simulink model "IEEE9_16b_central"  (R2020a)
settings: Solver=FixedStepAuto  StartTime=0.0  StopTime=5  FixedStep=1/1200/30  MaxStep=1e-4  RelTol=1e-3
undefined symbols (not defined in the file or in its folder): k
libraries: powerlib x33, powerlib_meascontrol x27, simulink_extras x24, dspsigops x6, sps_avr x3
(part 1 of 2)
settings Model: Creator=Pankaj  LastModifiedBy=ahmed
settings DataIOCC: ReturnWorkspaceOutputs=off  Refine=100
settings DebuggingCC: UnconnectedInputMsg=none  UnconnectedOutputMsg=none  UnconnectedLineMsg=none  ArithmeticOperatorsInVariantConditions=warning
settings SFSimCC: SimUseLocalCustomCode=off  CustomCodeUndefinedFunction=UseInterfaceOnly
settings RTWCC: RTWUseLocalCustomCode=off
settings CodeAppCC: StateflowObjectComments=on
settings SimscapeCC: SimscapeNormalizeSystem=off

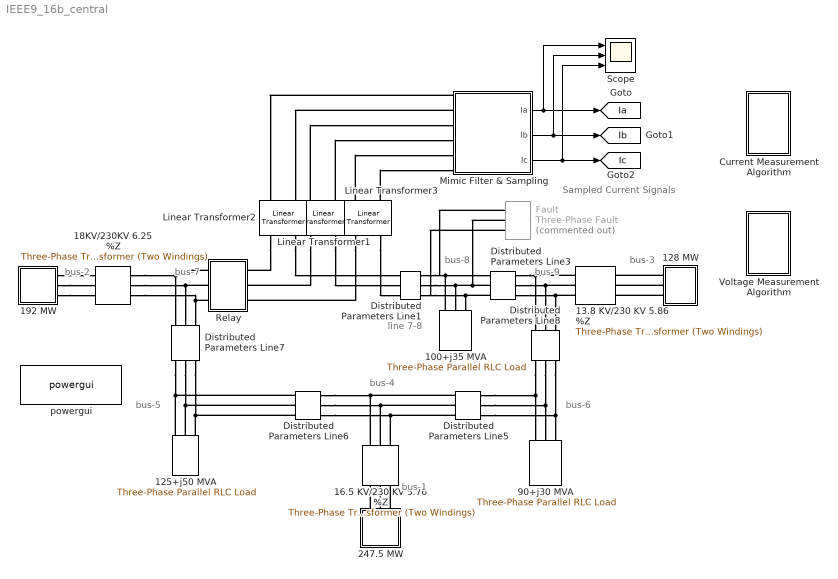
== system IEEE9_16b_central ==
  note: bus-2
  note: bus-7
  note: bus-8
  note: bus-9
  note: bus-1
  note: bus-3
  note: bus-4
  note: bus-6
  note: bus-5
  note: line 7-8
  note: Sampled Current Signals
  100+j35 MVA : powerlib/Elements/Three-Phase Parallel RLC Load  LConnTagsString=A|B|C  Configuration=Y (grounded)  NominalVoltage=(230000)*0.993698  Vabc=[1e3 1e3 1e3]  Vabcp=[1e3 1e3 1e3]  NominalFrequency=60  UnbalancedPower=off  ActivePower=100e6  InductivePower=35e6  CapacitivePower=0  Pabc=[10e3 9e3 11e3]  QLabc=[100 90 110]  QCabc=[100 90 110]  Pabcp=[10e3 9e3 11e3]  QLabcp=[100 90 110]  QCabcp=[100 90 110]  Measurements=None  LoadType=constant PQ
  125+j50 MVA : powerlib/Elements/Three-Phase Parallel RLC Load  LConnTagsString=A|B|C  Configuration=Y (grounded)  NominalVoltage=(223027)*1  Vabc=[1e3 1e3 1e3]  Vabcp=[1e3 1e3 1e3]  NominalFrequency=60  UnbalancedPower=off  ActivePower=125e6  InductivePower=50e6  CapacitivePower=0  Pabc=[10e3 9e3 11e3]  QLabc=[100 90 110]  QCabc=[100 90 110]  Pabcp=[10e3 9e3 11e3]  QLabcp=[100 90 110]  QCabcp=[100 90 110]  Measurements=None  LoadType=constant PQ
  128 MW : Subsystem
  13.8 KV/230 KV 5.86 %Z : powerlib/Elements/Three-Phase Transformer (Two Windings)  Winding1Connection=Yg  Winding2Connection=Yg  CoreType=Three single-phase transformers  SetSaturation=off  Hysteresis=off  DataFile='hysteresis'  SetInitialFlux=off  Measurements=None  UNITS=pu  NominalPower=[ 100e6 , 60 ]  Winding1=[13.8e3 , 1e-6 , 0 ]  Winding2=[ 230e3 , 1e-6, 0.0586 ]  Rm=500  Lm=500  L0=0.5  Saturation=[ 0,0 ; 0.0024,1.2 ; 1.0,1.52 ]  InitialFluxes=[ 0.8 , -0.8 , 0.7 ]  BreakLoop=off  DiscreteSolver=Trapezoidal iterative  DataType=off  TransfoNumber=1
  "16.5 KV/230 KV 5.76 %Z     " : powerlib/Elements/Three-Phase Transformer (Two Windings)  Winding1Connection=Yg  Winding2Connection=Yg  CoreType=Three single-phase transformers  SetSaturation=off  Hysteresis=off  DataFile='hysteresis'  SetInitialFlux=off  Measurements=None  UNITS=pu  NominalPower=[ 100e6 , 60 ]  Winding1=[16.5e3 , 1e-6, 0 ]  Winding2=[ 230e3 ,1e-6, 0.0576 ]  Rm=500  Lm=500  L0=0.5  Saturation=[ 0,0 ; 0.0024,1.2 ; 1.0,1.52 ]  InitialFluxes=[ 0.8 , -0.8 , 0.7 ]  BreakLoop=off  DiscreteSolver=Trapezoidal iterative  DataType=off  TransfoNumber=1
  18KV/230KV 6.25 %Z : powerlib/Elements/Three-Phase Transformer (Two Windings)  Winding1Connection=Yg  Winding2Connection=Yg  CoreType=Three single-phase transformers  SetSaturation=off  Hysteresis=off  DataFile='hysteresis'  SetInitialFlux=off  Measurements=None  UNITS=pu  NominalPower=[ 100e6 , 60 ]  Winding1=[ 18e3 , 1e-6 , 0]  Winding2=[ 230e3 , 1e-6, 0.0625 ]  Rm=500  Lm=500  L0=0.5  Saturation=[ 0,0 ; 0.0024,1.2 ; 1.0,1.52 ]  InitialFluxes=[ 0.8 , -0.8 , 0.7 ]  BreakLoop=off  DiscreteSolver=Trapezoidal iterative  DataType=off  TransfoNumber=1
  192 MW : Subsystem
  247.5 MW : Subsystem
  90+j30 MVA : powerlib/Elements/Three-Phase Parallel RLC Load  LConnTagsString=A|B|C  Configuration=Y (grounded)  NominalVoltage=(226177)*0.999999  Vabc=[1e3 1e3 1e3]  Vabcp=[1e3 1e3 1e3]  NominalFrequency=60  UnbalancedPower=off  ActivePower=90e6  InductivePower=30e6  CapacitivePower=0  Pabc=[10e3 9e3 11e3]  QLabc=[100 90 110]  QCabc=[100 90 110]  Pabcp=[10e3 9e3 11e3]  QLabcp=[100 90 110]  QCabcp=[100 90 110]  Measurements=None  LoadType=constant PQ
  Current Measurement Algorithm : Subsystem
  Distributed Parameters Line1 : powerlib/Elements/Distributed Parameters Line  Phases=3  Frequency=60  Resistance=[0.044965 0.11241]  Inductance="[1.01e-3  2.02e-3]"  Capacitance=[12.74e-9 7.751e-9]  Length=100  x1=[-0.000416666666666667 3.05242528703213e-10 0 0;-0.000388888888888889 3.05500631439883e-10 0 0;-0.000361111111111111 3.05725232589637e-10 75589.8043140482 -217739.673406231;-0.000333333333333333 3.05916307522428e-10 77865.7774864176 -216936.173033532;-0.000305555555555556 3.06073835284735e-10 80133.2117988181 -216108.883164811;-0.000277777777777778 3.06197798601864e-10 82391.8586015257 -215257.894521725;-0.00025 3.06288183879841e-10 84641.4702084657 -214383.30042477;-0.000222222222222222 3.06344981206902e-10 86881.7999243747 -213485.196783042;-0.000194444444444444 3.06368184354579e-10 89112.6020718531 -212563.682083727;-0.000166666666666667 3.06357790778386e-10 91333.6320183066 -211618.857381298;-0.000138888888888889 3.06313801618096e-10 93544.6462027728 -210650.826286428;-0.000111111111111111 3.06236221697615e-10 95745.4021626305 -209659.694954637;-8.33333333333333e-05 3.06125059524457e-10 97935.6585601885 -208645.572074645;-5.55555555555556e-05 3.05980327288806e-10 100115.175209151 -207608.568856452;-2.77777777777778e-05 3.05802040862183e-10 102283.713100956 -206548.799019148]  x2=[-0.000416666666666667 1.02171489544743e-10 0 0;-0.000388888888888889 1.0125535769788e-10 0 0;-0.000361111111111111 1.00328122060001e-10 65357.6959924733 -218991.76000131;-0.000333333333333333 9.93898843129427e-11 67647.34161361 -218295.340188402;-0.000305555555555556 9.84407473450475e-11 69929.5689414224 -217574.981831478;-0.000277777777777778 9.74808152398795e-11 72204.1277039659 -216830.763925948;-0.00025 9.65101932648115e-11 74470.76847024 -216062.768083693;-0.000222222222222222 9.55289878594811e-11 76729.2426775421 -215271.078524112;-0.000194444444444444 9.45373066241179e-11 78979.3026587246 -214455.782064886;-0.000166666666666667 9.35352583077448e-11 81220.7016693547 -213616.96811246;-0.000138888888888889 9.25229527962518e-11 83453.1939147727 -212754.728652235;-0.000111111111111111 9.15005011003457e-11 85676.5345770459 -211869.158238486;-8.33333333333333e-05 9.0468015343377e-11 87890.4798418159 -210960.353983988;-5.55555555555556e-05 8.94256087490441e-11 90094.7869250356 -210028.415549369;-2.77777777777778e-05 8.83733956289768e-11 92289.214099593 -209073.445132179]  x3=[-0.000416666666666667 1.88047725229952e-12 0 0;-0.000388888888888889 1.85577565108302e-12 0 0;-0.000361111111111111 1.83087054315368e-12 150.014670555124 -522.196921384387;-0.000333333333333333 1.80576465963726e-12 155.474780219226 -520.59737046614;-0.000305555555555556 1.78046075367679e-12 160.917840321636 -518.940730179622;-0.000277777777777778 1.75496160013071e-12 166.343253969475 -517.227182194109;-0.00025 1.72926999526855e-12 171.750426204999 -515.456914419448;-0.000222222222222222 1.70338875646432e-12 177.138764070837 -513.63012098545;-0.000194444444444444 1.67732072188749e-12 182.507676675023 -511.7470022206;-0.000166666666666667 1.65106875019181e-12 187.856575255787 -509.807764630092;-0.000138888888888889 1.62463572020183e-12 193.184873246123 -507.812620873181;-0.000111111111111111 1.59802453059714e-12 198.491986338112 -505.761789739863;-8.33333333333333e-05 1.57123809959458e-12 203.777332546997 -503.655496126883;-5.55555555555556e-05 1.54427936462815e-12 209.040332275007 -501.493971013071;-2.77777777777778e-05 1.51715128202694e-12 214.280408374913 -499.277451434014]  x4=[-0.000416666666666667 -8.7518100237193e-13 0 0;-0.000388888888888889 -8.47376987953706e-13 0 0;-0.000361111111111111 -8.19480049099682e-13 240.406666770988 -1044.04487087356;-0.000333333333333333 -7.91493245023573e-13 251.326459490831 -1041.47013077654;-0.000305555555555556 -7.6341964479383e-13 262.218691432199 -1038.78118174338;-0.000277777777777778 -7.35262326997077e-13 273.082168139116 -1035.97831864764;-0.00025 -7.07024379400516e-13 283.915698308939 -1033.06184885485;-0.000222222222222222 -6.78708898613313e-13 294.718093923004 -1030.03209218878;-0.000194444444444444 -6.50318989747023e-13 305.488170376899 -1026.88938089639;-0.000166666666666667 -6.21857766075078e-13 316.224746610374 -1023.6340596114;-0.000138888888888889 -5.93328348691383e-13 326.926645236854 -1020.26648531647;-0.000111111111111111 -5.64733866168052e-13 337.592692672555 -1016.78702730406;-8.33333333333333e-05 -5.36077454212322e-13 348.221719265181 -1013.19606713596;-5.55555555555556e-05 -5.07362255322695e-13 358.812559422187 -1009.49399860142;-2.77777777777778e-05 -4.78591418444318e-13 369.364051738602 -1005.68122767396]  x5=0.000395689524753941  V1=[5.416e-10 2.305e+05 2.305e+05;377 377 377;2.885 0.3359 -1.235]  V2=[2.789e-10 2.285e+05 2.285e+05;377 377 377;2.728 0.2916 -1.279]  I1=[3.179e-12 542 542;377 377 377;-1.76 0.2811 -1.29]  I2=[4.124e-12 1072 1072;377 377 377;1.614 0.2282 -1.343]  nHarmo=1  Measurements=None
  Distributed Parameters Line3 : powerlib/Elements/Distributed Parameters Line  Phases=3  Frequency=60  Resistance=[ 0.062951 0.15737]  Inductance="[ 1.414e-3  3.53e-3]"  Capacitance=[12.74e-9 7.751e-9]  Length=100  x1=[-0.000527777777777778 1.05722988233672e-10 0 0;-0.0005 1.04852263851676e-10 0 0;-0.000472222222222222 1.03970041237372e-10 0 0;-0.000444444444444444 1.0307641713641e-10 58446.7641257665 -220936.637648747;-0.000416666666666667 1.02171489544743e-10 60757.1549979699 -220312.481147461;-0.000388888888888889 1.0125535769788e-10 63060.8831634568 -219664.164899921;-0.000361111111111111 1.00328122060001e-10 65357.6959924733 -218991.76000131;-0.000333333333333333 9.93898843129427e-11 67647.34161361 -218295.340188402;-0.000305555555555556 9.84407473450475e-11 69929.5689414224 -217574.981831478;-0.000277777777777778 9.74808152398795e-11 72204.1277039659 -216830.763925948;-0.00025 9.65101932648115e-11 74470.76847024 -216062.768083693;-0.000222222222222222 9.55289878594811e-11 76729.2426775421 -215271.078524112;-0.000194444444444444 9.45373066241179e-11 78979.3026587246 -214455.782064886;-0.000166666666666667 9.35352583077448e-11 81220.7016693547 -213616.96811246;-0.000138888888888889 9.25229527962518e-11 83453.1939147727 -212754.728652235;-0.000111111111111111 9.15005011003457e-11 85676.5345770459 -211869.158238486;-8.33333333333333e-05 9.0468015343377e-11 87890.4798418159 -210960.353983988;-5.55555555555556e-05 8.94256087490441e-11 90094.7869250356 -210028.415549369;-2.77777777777778e-05 8.83733956289768e-11 92289.214099593 -209073.445132179]  x2=[-0.000527777777777778 9.13415239263644e-11 0 0;-0.0005 9.12184788255193e-11 0 0;-0.000472222222222222 9.10854305905322e-11 0 0;-0.000444444444444444 9.09423938116413e-11 67569.0569929193 -221221.006139122;-0.000416666666666667 9.07893841744413e-11 69881.9252697332 -220501.30792954;-0.000388888888888889 9.06264184581633e-11 72187.1302059435 -219757.42926672;-0.000361111111111111 9.04535145338344e-11 74484.4190098517 -218989.451725339;-0.000333333333333333 9.02706913623184e-11 76773.5397578524 -218197.45952279;-0.000305555555555556 9.00779689922363e-11 79054.2414220595 -217381.539509942;-0.000277777777777778 8.98753685577677e-11 81326.2738978343 -216541.78116162;-0.00025 8.96629122763335e-11 83589.3880312124 -215678.276566789;-0.000222222222222222 8.9440623446159e-11 85843.3356462261 -214791.120418459;-0.000194444444444444 8.92085264437193e-11 88087.8695721197 -213880.4100033;-0.000166666666666667 8.89666467210664e-11 90322.7436704547 -212946.24519097;-0.000138888888888889 8.87150108030376e-11 92547.7128621014 -211988.72842317;-0.000111111111111111 8.84536462843469e-11 94762.5331541149 -211007.964702401;-8.33333333333333e-05 8.81825818265591e-11 96966.9616664913 -210004.06158046;-5.55555555555556e-05 8.79018471549467e-11 99160.7566588026 -208977.129146636;-2.77777777777778e-05 8.76114730552299e-11 101343.677556706 -207927.280015642]  x3=[-0.000527777777777778 -5.71619859169204e-13 0 0;-0.0005 -5.80597990208738e-13 0 0;-0.000472222222222222 -5.89512452135901e-13 0 0;-0.000444444444444444 -5.98362267379486e-13 134.783300599734 -836.294175870902;-0.000416666666666667 -6.07146465457522e-13 143.533396667207 -834.836905447173;-0.000388888888888889 -6.15864083083703e-13 152.267752680261 -833.288085749006;-0.000361111111111111 -6.24514164273016e-13 160.985410818333 -831.647886621933;-0.000333333333333333 -6.33095760446581e-13 169.685415091968 -829.916487932272;-0.000305555555555556 -6.41607930535672e-13 178.366811447656 -828.0940795474;-0.000277777777777778 -6.50049741084917e-13 187.028647872459 -826.180861314934;-0.00025 -6.58420266354656e-13 195.669974498401 -824.177043040813;-0.000222222222222222 -6.66718588422468e-13 204.289843706639 -822.082844466291;-0.000194444444444444 -6.74943797283823e-13 212.887310231377 -819.898495243842;-0.000166666666666667 -6.83094990951881e-13 221.461431263526 -817.624234911973;-0.000138888888888889 -6.91171275556401e-13 230.011266554094 -815.260312868959;-0.000111111111111111 -6.99171765441763e-13 238.535878517293 -812.806988345489;-8.33333333333333e-05 -7.07095583264095e-13 247.034332333357 -810.264530376245;-5.55555555555556e-05 -7.14941860087479e-13 255.505696051058 -807.633217770394;-2.77777777777778e-05 -7.22709735479242e-13 263.949040689898 -804.913339081016]  x4=[-0.000527777777777778 6.12064546598544e-13 0 0;-0.0005 6.08521806486011e-13 0 0;-0.000472222222222222 6.04912335099979e-13 0 0;-0.000444444444444444 6.01236528259661e-13 132.734580460085 -502.248002708346;-0.000416666666666667 5.974947890587e-13 137.986709125664 -500.830491731963;-0.000388888888888889 5.93687527820964e-13 143.223705993618 -499.358059048314;-0.000361111111111111 5.89815162055552e-13 148.444996768225 -497.830866126237;-0.000333333333333333 5.85878116411009e-13 153.650008876114 -496.249080439645;-0.000305555555555556 5.81876822628754e-13 158.838171529051 -494.612875449165;-0.000277777777777778 5.77811719495742e-13 164.008915786537 -492.92243058311;-0.00025 5.73683252796342e-13 169.161674618194 -491.177931217812;-0.000222222222222222 5.69491875263449e-13 174.29588296595 -489.379568657283;-0.000194444444444444 5.65238046528844e-13 179.410977806003 -487.527540112244;-0.000166666666666667 5.60922233072783e-13 184.506398210562 -485.622048678496;-0.000138888888888889 5.56544908172847e-13 189.581585409359 -483.663303314648;-0.000111111111111111 5.52106551852038e-13 194.635982850925 -481.651518819201;-8.33333333333333e-05 5.47607650826144e-13 199.669036263624 -479.586915806996;-5.55555555555556e-05 5.43048698450359e-13 204.680193716431 -477.469720685019;-2.77777777777778e-05 5.38430194665186e-13 209.66890567946 -475.300165627575]  x5=0.000523077718890797  V1=[2.541e-10 2.285e+05 2.285e+05;377 377 377;2.713 0.2668 -1.304]  V2=[4.31e-10 2.313e+05 2.313e+05;377 377 377;2.564 0.3044 -1.266]  I1=[1.418e-12 846 846;377 377 377;1.513 0.1676 -1.403]  I2=[2.062e-12 520.4 520.5;377 377 377;-2.991 0.2668 -1.304]  nHarmo=1  Measurements=None
  Distributed Parameters Line5 : powerlib/Elements/Distributed Parameters Line  Phases=3  Frequency=60  Resistance=[ 0.08993 0.224825]  Inductance="[ 1.29e-3  3.22e-3]"  Capacitance=[12.74e-9 7.751e-9]  Length=100  x1=[-0.0005 1.84418084980096e-10 59301.0004761159 -221128.521904105;-0.000472222222222222 1.86482822406443e-10 61613.3539298093 -220495.408761845;-0.000444444444444444 1.88527109889844e-10 63918.9507849249 -219838.115813256;-0.000416666666666667 1.90550723251138e-10 66217.5382067858 -219156.715137918;-0.000388888888888889 1.92553440578315e-10 68508.8641293785 -218451.281459093;-0.000361111111111111 1.94535042250854e-10 70792.6772829948 -217721.892135534;-0.000333333333333333 1.96495310963798e-10 73068.7272217859 -216968.627152999;-0.000305555555555556 1.98434031751595e-10 75336.7643512275 -216191.569115483;-0.000277777777777778 2.00350992011662e-10 77596.5399554898 -215390.803236157;-0.00025 2.02245981527704e-10 79847.8062247124 -214566.417328021;-0.000222222222222222 2.04118792492767e-10 82090.3162821795 -213718.501794282;-0.000194444444444444 2.05969219532023e-10 84323.8242113925 -212847.149618432;-0.000166666666666667 2.07797059725295e-10 86548.0850830376 -211952.456354057;-0.000138888888888889 2.09602112629309e-10 88762.8549818451 -211034.520114356;-0.000111111111111111 2.11384180299671e-10 90967.8910333373 -210093.441561382;-8.33333333333333e-05 2.13143067312581e-10 93162.9514304628 -209129.323895003;-5.55555555555556e-05 2.14878580786255e-10 95347.7954601129 -208142.272841585;-2.77777777777778e-05 2.16590530402085e-10 97522.1835295188 -207132.3966424]  x2=[-0.0005 1.973914942299e-10 47829.0767997227 -221055.102399272;-0.000472222222222222 1.97930112644823e-10 50141.2903619321 -220542.12557881;-0.000444444444444444 1.98447025792425e-10 52448.0053666123 -220004.963828994;-0.000416666666666667 1.98942176987354e-10 54748.9688564689 -219443.676055664;-0.000388888888888889 1.99415511930702e-10 57043.9285049254 -218858.323810348;-0.000361111111111111 1.99866978715958e-10 59332.6326437948 -218248.971283518;-0.000333333333333333 2.00296527834702e-10 61614.8302908768 -217615.685297545;-0.000305555555555556 2.00704112182032e-10 63890.2711774814 -216958.535299372;-0.000277777777777778 2.01089687061731e-10 66158.7057758734 -216277.593352903;-0.00025 2.0145321019117e-10 68419.8853266363 -215572.934131097;-0.000222222222222222 2.01794641705939e-10 70673.5618659511 -214844.634907777;-0.000194444444444444 2.02113944164227e-10 72919.4882527886 -214092.77554916;-0.000166666666666667 2.02411082550919e-10 75157.4181960113 -213317.438505097;-0.000138888888888889 2.02686024281445e-10 77387.1062813816 -212518.708800034;-0.000111111111111111 2.02938739205344e-10 79608.3079984748 -211696.674023683;-8.33333333333333e-05 2.03169199609578e-10 81820.7797674918 -210851.42432142;-5.55555555555556e-05 2.03377380221565e-10 84024.278965971 -209983.052384401;-2.77777777777778e-05 2.03563258211957e-10 86218.563955394 -209091.653439394]  x3=[-0.0005 1.45931914328997e-12 89.8864515456847 -468.322639248616;-0.000472222222222222 1.46185650921508e-12 94.7856956152835 -467.355690941637;-0.000444444444444444 1.46423356610033e-12 99.6745453652203 -466.337491816527;-0.000416666666666667 1.46645005327464e-12 104.552464678028 -465.268153530294;-0.000388888888888889 1.46850572767522e-12 109.418918634884 -464.14779334793;-0.000361111111111111 1.47040036387421e-12 114.273373574273 -462.976534129555;-0.000333333333333333 1.47213375410339e-12 119.115297150506 -461.754504316942;-0.000305555555555556 1.47370570827699e-12 123.944158392098 -460.48183791943;-0.000277777777777778 1.47511605401253e-12 128.75942776 -459.158674499231;-0.00025 1.4763646366497e-12 133.56057720566 -457.785159156126;-0.000222222222222222 1.47745131926734e-12 138.347080228939 -456.36144251155;-0.000194444444444444 1.47837598269846e-12 143.118411935841 -454.887680692075;-0.000166666666666667 1.4791385255433e-12 147.874049096077 -453.364035312295;-0.000138888888888889 1.47973886418043e-12 152.613470200439 -451.790673457095;-0.000111111111111111 1.48017693277596e-12 157.336155517997 -450.167767663332;-8.33333333333333e-05 1.48045268329074e-12 162.041587153085 -448.495495900915;-5.55555555555556e-05 1.48056608548561e-12 166.729249102099 -446.774041553287;-2.77777777777778e-05 1.48051712692474e-12 171.398627310082 -445.003593397318]  x4=[-0.0005 -9.64211279668315e-13 134.813064300476 -917.533563496279;-0.000472222222222222 -9.64297994881882e-13 144.413854297421 -916.071516812538;-0.000444444444444444 -9.64278963953659e-13 153.998807687847 -914.509012563791;-0.000416666666666667 -9.64154188970602e-13 163.5668733736 -912.846222096237;-0.000388888888888889 -9.63923683615695e-13 173.117002108457 -911.083327753587;-0.000361111111111111 -9.63587473166446e-13 182.648146613182 -909.220522857074;-0.000333333333333333 -9.63145594492122e-13 192.159261690373 -907.258011684245;-0.000305555555555556 -9.62598096049696e-13 201.649304339081 -905.196009446567;-0.000277777777777778 -9.61945037878544e-13 211.117233869188 -903.03474226582;-0.00025 -9.61186491593854e-13 220.562012015526 -900.774447149308;-0.000222222222222222 -9.60322540378773e-13 229.982603051738 -898.415371963861;-0.000194444444444444 -9.59353278975288e-13 239.377973903858 -895.957775408657;-0.000166666666666667 -9.58278813673834e-13 248.747094263594 -893.401926986852;-0.000138888888888889 -9.57099262301641e-13 258.088936701319 -890.748106976029;-0.000111111111111111 -9.55814754209808e-13 267.402476778737 -887.996606397457;-8.33333333333333e-05 -9.54425430259122e-13 276.686693161225 -885.147726984182;-5.55555555555556e-05 -9.52931442804611e-13 285.940567729831 -882.201781147934;-2.77777777777778e-05 -9.51332955678836e-13 295.163085692929 -879.159091944873]  x5=0.000499582025297148  V1=[3.29e-10 2.289e+05 2.289e+05;377 377 377;2.341 0.2974 -1.273]  V2=[3.35e-10 2.261e+05 2.261e+05;377 377 377;2.353 0.2487 -1.322]  I1=[9.5e-13 477.9 477.9;377 377 377;2.529 0.2254 -1.345]  I2=[6.245e-14 926.2 926.2;377 377 377;-2.223 0.1812 -1.39]  nHarmo=1  Measurements=None
  Distributed Parameters Line6 : powerlib/Elements/Distributed Parameters Line  Phases=3  Frequency=60  Resistance=[ 0.0529 0.13225]  Inductance="[ 1.192e-3  2.38e-3]"  Capacitance=[12.74e-9 7.751e-9]  Length=100  x1=[-0.000444444444444444 2.52199341782817e-10 0 0;-0.000416666666666667 2.53018573393811e-10 51153.0343164036 -217071.620180754;-0.000388888888888889 2.53810058666972e-10 53423.351654107 -216524.053460858;-0.000361111111111111 2.5457371080702e-10 55687.8105192751 -215952.742438496;-0.000333333333333333 2.55309446070894e-10 57946.1625884752 -215357.749764359;-0.000305555555555556 2.5601718377693e-10 60198.1602079536 -214739.1406861;-0.000277777777777778 2.56696846313713e-10 62443.5564207935 -214096.983041174;-0.00025 2.57348359148588e-10 64682.104993997 -213431.347249403;-0.000222222222222222 2.57971650835829e-10 66913.5604454869 -212742.306305254;-0.000194444444444444 2.5856665302448e-10 69137.6780710265 -212029.935769831;-0.000166666666666667 2.59133300465846e-10 71354.213971055 -211294.313762591;-0.000138888888888889 2.59671531020649e-10 73562.9250774325 -210535.520952776;-0.000111111111111111 2.60181285665843e-10 75763.5691800965 -209753.640550569;-8.33333333333333e-05 2.60662508501087e-10 77955.9049536221 -208948.758297966;-5.55555555555556e-05 2.61115146754875e-10 80139.6919836863 -208120.962459378;-2.77777777777778e-05 2.6153915079032e-10 82314.6907934322 -207270.343811946]  x2=[-0.000444444444444444 1.88527109889844e-10 0 0;-0.000416666666666667 1.90550723251138e-10 66217.5382067858 -219156.715137918;-0.000388888888888889 1.92553440578315e-10 68508.8641293785 -218451.281459093;-0.000361111111111111 1.94535042250854e-10 70792.6772829948 -217721.892135534;-0.000333333333333333 1.96495310963798e-10 73068.7272217859 -216968.627152999;-0.000305555555555556 1.98434031751595e-10 75336.7643512275 -216191.569115483;-0.000277777777777778 2.00350992011662e-10 77596.5399554898 -215390.803236157;-0.00025 2.02245981527704e-10 79847.8062247124 -214566.417328021;-0.000222222222222222 2.04118792492767e-10 82090.3162821795 -213718.501794282;-0.000194444444444444 2.05969219532023e-10 84323.8242113925 -212847.149618432;-0.000166666666666667 2.07797059725295e-10 86548.0850830376 -211952.456354057;-0.000138888888888889 2.09602112629309e-10 88762.8549818451 -211034.520114356;-0.000111111111111111 2.11384180299671e-10 90967.8910333373 -210093.441561382;-8.33333333333333e-05 2.13143067312581e-10 93162.9514304628 -209129.323895003;-5.55555555555556e-05 2.14878580786255e-10 95347.7954601129 -208142.272841585;-2.77777777777778e-05 2.16590530402085e-10 97522.1835295188 -207132.3966424]  x3=[-0.000444444444444444 -1.01163623569235e-12 0 0;-0.000416666666666667 -1.01948713157847e-12 106.317395247665 -1047.05010725269;-0.000388888888888889 -1.02722622921203e-12 117.276022997576 -1045.8793627485;-0.000361111111111111 -1.03485267991377e-12 128.221790109984 -1044.59392578619;-0.000333333333333333 -1.04236564735742e-12 139.153496258179 -1043.19393732841;-0.000305555555555556 -1.04976430766146e-12 150.069942657391 -1041.67955089968;-0.000277777777777778 -1.05704784947938e-12 160.969932196256 -1040.05093256953;-0.00025 -1.06421547408877e-12 171.85226956809 -1038.30826093431;-0.000222222222222222 -1.0712663954788e-12 182.715761401967 -1036.45172709761;-0.000194444444444444 -1.0781998404365e-12 193.559216393586 -1034.48153464929;-0.000166666666666667 -1.08501504863148e-12 204.381445435914 -1032.39789964315;-0.000138888888888889 -1.09171127269937e-12 215.18126174958 -1030.20105057324;-0.000111111111111111 -1.09828777832375e-12 225.957481013023 -1027.89122834883;-8.33333333333333e-05 -1.10474384431665e-12 236.708921492364 -1025.46868626795;-5.55555555555556e-05 -1.11107876269769e-12 247.434404170995 -1022.93368998963;-2.77777777777778e-05 -1.11729183877168e-12 258.132752878878 -1020.2865175048]  x4=[-0.000444444444444444 1.40469739549799e-12 0 0;-0.000416666666666667 1.41993404758416e-12 168.402373729606 -388.679228665907;-0.000388888888888889 1.43501498790081e-12 172.463297114689 -386.8944397103;-0.000361111111111111 1.44993856265288e-12 176.50530795576 -385.067223419474;-0.000333333333333333 1.46470313530224e-12 180.527963000778 -383.197780168287;-0.000305555555555556 1.47930708674711e-12 184.530821120289 -381.286314962258;-0.000277777777777778 1.49374881549964e-12 188.51344335579 -379.333037415088;-0.00025 1.50802673786154e-12 192.475392967874 -377.33816172567;-0.000222222222222222 1.5221392880977e-12 196.416235484119 -375.301906654604;-0.000194444444444444 1.53608491860798e-12 200.335538746733 -373.224495500205;-0.000166666666666667 1.54986210009683e-12 204.232872959947 -371.106156074017;-0.000138888888888889 1.56346932174105e-12 208.107810737146 -368.94712067583;-0.000111111111111111 1.57690509135544e-12 211.959927147735 -366.747626068204;-8.33333333333333e-05 1.59016793555646e-12 215.788799763742 -364.507913450509;-5.55555555555556e-05 1.60325639992377e-12 219.594008706135 -362.228228432474;-2.77777777777778e-05 1.61616904915978e-12 223.375136690875 -359.90882100725]  x5=0.000429504132692574  V1=[5.692e-10 2.23e+05 2.23e+05;377 377 377;2.022 0.2411 -1.33]  V2=[3.29e-10 2.289e+05 2.289e+05;377 377 377;2.367 0.3033 -1.267]  I1=[3.839e-12 1053 1053;377 377 377;3.112 0.1114 -1.459]  I2=[2.337e-12 422.3 422.3;377 377 377;0.2722 0.4185 -1.152]  nHarmo=1  Measurements=None
  Distributed Parameters Line7 : powerlib/Elements/Distributed Parameters Line  Phases=3  Frequency=60  Resistance=[ 0.16928 0.4232]  Inductance="[ 2.259e-3  5.64e-3]"  Capacitance=[12.74e-9 7.751e-9]  Length=100  x1=[-0.000666666666666667 2.30563295499809e-10 30497.8167078401 -220922.18353086;-0.000638888888888889 2.31563886547772e-10 32809.5887794555 -220590.703141853;-0.000611111111111111 2.32539084006088e-10 35117.7629099308 -220235.032496416;-0.000583333333333333 2.33488780933365e-10 37422.0859819617 -219855.210597842;-0.000555555555555556 2.34412873184633e-10 39722.3053005562 -219451.279097883;-0.000527777777777778 2.35311259422764e-10 42018.1686207448 -219023.28229218;-0.0005 2.36183841129582e-10 44309.4241752423 -218571.267115405;-0.000472222222222222 2.3703052261667e-10 46595.8207020573 -218095.283136117;-0.000444444444444445 2.37851211035862e-10 48877.1074720451 -217595.382551323;-0.000416666666666667 2.38645816389424e-10 51153.0343164036 -217071.620180754;-0.000388888888888889 2.39414251539926e-10 53423.351654107 -216524.053460858;-0.000361111111111111 2.40156432219792e-10 55687.8105192751 -215952.742438496;-0.000333333333333333 2.40872277040549e-10 57946.1625884753 -215357.749764359;-0.000305555555555556 2.41561707501745e-10 60198.1602079536 -214739.1406861;-0.000277777777777778 2.42224647999559e-10 62443.5564207936 -214096.983041174;-0.00025 2.42861025835097e-10 64682.1049939971 -213431.347249403;-0.000222222222222222 2.43470771222358e-10 66913.5604454869 -212742.306305254;-0.000194444444444444 2.44053817295887e-10 69137.6780710266 -212029.935769831;-0.000166666666666667 2.44610100118114e-10 71354.213971055 -211294.313762591;-0.000138888888888889 2.45139558686357e-10 73562.9250774325 -210535.520952776;-0.000111111111111111 2.45642134939518e-10 75763.5691800965 -209753.640550569;-8.33333333333333e-05 2.46117773764448e-10 77955.9049536221 -208948.758297966;-5.55555555555556e-05 2.4656642300199e-10 80139.6919836863 -208120.962459378;-2.77777777777778e-05 2.46988033452698e-10 82314.6907934323 -207270.343811946]  x2=[-0.000666666666666667 3.10465197724416e-10 50471.8328539013 -224882.541473884;-0.000638888888888889 3.10653612663979e-10 52823.9817050564 -224341.679984892;-0.000611111111111111 3.10807960934166e-10 55170.3378113455 -223776.216902588;-0.000583333333333333 3.10928225608948e-10 57510.6438683803 -223186.214236372;-0.000555555555555556 3.1101439349995e-10 59844.6432352289 -222571.736686685;-0.000527777777777778 3.11066455157891e-10 62172.0799625589 -221932.851637915;-0.0005 3.11084404873623e-10 64492.6988207054 -221269.629151007;-0.000472222222222222 3.11068240678759e-10 66806.2453276595 -220582.141955781;-0.000444444444444445 3.11017964345883e-10 69112.4657769755 -219870.465442954;-0.000416666666666667 3.10933581388364e-10 71411.1072655924 -219134.677655876;-0.000388888888888889 3.10815101059742e-10 73701.9177215675 -218374.85928197;-0.000361111111111111 3.10662536352721e-10 75984.6459317193 -217591.093643883;-0.000333333333333333 3.1047590399774e-10 78259.0415691756 -216783.466690349;-0.000305555555555556 3.1025522446114e-10 80524.8552208246 -215952.066986765;-0.000277777777777778 3.1000052194292e-10 82781.838414666 -215096.985705477;-0.00025 3.0971182437408e-10 85029.7436470587 -214218.316615784;-0.000222222222222222 3.09389163413563e-10 87268.3244098624 -213316.156073652;-0.000194444444444444 3.09032574444779e-10 89497.3352174699 -212390.603011153;-0.000166666666666667 3.08642096571726e-10 91716.5316337275 -211441.758925609;-0.000138888888888889 3.08217772614703e-10 93925.6702987401 -210469.727868467;-0.000111111111111111 3.07759649105615e-10 96124.5089555584 -209474.616433886;-8.33333333333333e-05 3.07267776282866e-10 98312.8064767449 -208456.533747048;-5.55555555555556e-05 3.06742208085855e-10 100490.322890817 -207415.591452194;-2.77777777777778e-05 3.06183002149057e-10 102656.81940856 -206351.903700375]  x3=[-0.000666666666666667 3.95193425002914e-13 17.8156603133809 -747.671231727835;-0.000638888888888889 3.97733065716012e-13 25.6441190782873 -747.443674381332;-0.000611111111111111 4.0022909051641e-13 33.4697656765538 -747.134151413007;-0.000583333333333333 4.02681225686861e-13 41.2917419378438 -746.742696765544;-0.000555555555555556 4.05089202323111e-13 49.1091900943147 -746.269353366355;-0.000527777777777778 4.07452756363385e-13 56.9212528746816 -745.714173122878;-0.0005 4.09771628617349e-13 64.7270735982265 -745.077216916883;-0.000472222222222222 4.12045564794528e-13 72.5257962687434 -744.358554597796;-0.000444444444444445 4.14274315532196e-13 80.3165656684082 -743.55826497504;-0.000416666666666667 4.16457636422719e-13 88.0985274515619 -742.676435809388;-0.000388888888888889 4.18595288040357e-13 95.8708282384004 -741.713163803348;-0.000361111111111111 4.20687035967521e-13 103.632615708557 -740.668554590548;-0.000333333333333333 4.2273265082048e-13 111.383038694567 -739.542722724162;-0.000305555555555556 4.24731908274512e-13 119.121247275211 -738.33579166434;-0.000277777777777778 4.26684589088508e-13 126.846392868718 -737.047893764674;-0.00025 4.28590479129012e-13 134.557628325817 -735.679170257682;-0.000222222222222222 4.30449369393705e-13 142.254108022644 -734.22977123932;-0.000194444444444444 4.32261056034319e-13 149.934987953468 -732.699855652525;-0.000166666666666667 4.34025340379e-13 157.59942582325 -731.08959126978;-0.000138888888888889 4.35742028954088e-13 165.246581140005 -729.399154674722;-0.000111111111111111 4.37410933505334e-13 172.875615306979 -727.628731242772;-8.33333333333333e-05 4.39031871018548e-13 180.485691714604 -725.778515120811;-5.55555555555556e-05 4.40604663739666e-13 188.075975832243 -723.848709205887;-2.77777777777778e-05 4.42129139194241e-13 195.645635299708 -721.839525122964]  x4=[-0.000666666666666667 -2.54027812318938e-14 63.4642635309681 -298.647101139942;-0.000638888888888889 -2.78676951249853e-14 66.588143768232 -297.966141505749;-0.000611111111111111 -3.03295530112661e-14 69.7047218651515 -297.252506526367;-0.000583333333333333 -3.27880849202761e-14 72.8136560538176 -296.506274459913;-0.000555555555555556 -3.52430212462865e-14 75.9146054045622 -295.727527139143;-0.000527777777777778 -3.76940927778645e-14 79.0072298633443 -294.916349962475;-0.0005 -4.01410307273956e-14 82.0911902890413 -294.072831884629;-0.000472222222222222 -4.25835667605591e-14 85.1661484906394 -293.197065406867;-0.000444444444444445 -4.50214330257542e-14 88.2317672643203 -292.289146566853;-0.000416666666666667 -4.74543621834725e-14 91.2877104304391 -291.349174928118;-0.000388888888888889 -4.98820874356154e-14 94.3336428703901 -290.377253569146;-0.000361111111111111 -5.23043425547509e-14 97.3692305633569 -289.373489072065;-0.000333333333333333 -5.47208619133089e-14 100.394140622941 -288.337991510965;-0.000305555555555556 -5.71313805127101e-14 103.408041333666 -287.270874439822;-0.000277777777777778 -5.95356340124259e-14 106.410602187357 -286.172254880049;-0.00025 -6.19333587589666e-14 109.401493919379 -285.042253307659;-0.000222222222222222 -6.43242918147939e-14 112.380388544751 -283.88099364006;-0.000194444444444444 -6.67081709871548e-14 115.346959394106 -282.68860322246;-0.000166666666666667 -6.90847348568342e-14 118.300881149522 -281.465212813906;-0.000138888888888889 -7.14537228068224e-14 121.24182988019 -280.210956572942;-0.000111111111111111 -7.38148750508945e-14 124.16948307794 -278.9259720429;-8.33333333333333e-05 -7.61679326620992e-14 127.083519692608 -277.610400136813;-5.55555555555556e-05 -7.8512637601153e-14 129.983620167241 -276.264385121966;-2.77777777777778e-05 -8.08487327447368e-14 132.86946647314 -274.888074604073]  x5=0.000661178039562719  V1=[5.692e-10 2.23e+05 2.23e+05;377 377 377;1.934 0.1858 -1.385]  V2=[7.107e-10 2.305e+05 2.305e+05;377 377 377;2.15 0.2689 -1.302]  I1=[1.362e-12 746.7 746.7;377 377 377;1.537 0.07174 -1.499]  I2=[6.286e-13 306.4 306.4;377 377 377;-2.668 0.2582 -1.313]  nHarmo=1  Measurements=None
  Distributed Parameters Line8 : powerlib/Elements/Distributed Parameters Line  Phases=3  Frequency=60  Resistance=[ 0.20631 0.5157]  Inductance="[ 2.38e-3  6.09e-3]"  Capacitance=[12.74e-9 7.751e-9]  Length=100  x1=[-0.000694444444444444 2.07074748311912e-10 0 0;-0.000666666666666667 2.07802186629336e-10 0 0;-0.000638888888888889 2.08506837095279e-10 0 0;-0.000611111111111111 2.09188622436875e-10 0 0;-0.000583333333333333 2.0984746788868e-10 0 0;-0.000555555555555556 2.10483301200865e-10 43189.1688189828 -222008.278895698;-0.000527777777777778 2.11096052647142e-10 45511.6182402574 -221543.838036691;-0.0005 2.1168565503241e-10 47829.0767997227 -221055.102399272;-0.000472222222222222 2.12252043700123e-10 50141.2903619321 -220542.12557881;-0.000444444444444444 2.12795156539381e-10 52448.0053666123 -220004.963828994;-0.000416666666666667 2.13314933991741e-10 54748.9688564689 -219443.676055664;-0.000388888888888889 2.13811319057748e-10 57043.9285049254 -218858.323810348;-0.000361111111111111 2.14284257303186e-10 59332.6326437948 -218248.971283518;-0.000333333333333333 2.14733696865047e-10 61614.8302908768 -217615.685297545;-0.000305555555555556 2.15159588457217e-10 63890.2711774814 -216958.535299372;-0.000277777777777778 2.15561885375885e-10 66158.7057758734 -216277.593352903;-0.00025 2.1594054350466e-10 68419.8853266363 -215572.934131097;-0.000222222222222222 2.16295521319411e-10 70673.5618659511 -214844.634907777;-0.000194444444444444 2.1662677989282e-10 72919.4882527886 -214092.77554916;-0.000166666666666667 2.16934282898652e-10 75157.4181960113 -213317.438505097;-0.000138888888888889 2.17217996615737e-10 77387.1062813816 -212518.708800034;-0.000111111111111111 2.17477889931669e-10 79608.3079984748 -211696.674023683;-8.33333333333333e-05 2.17713934346216e-10 81820.7797674918 -210851.42432142;-5.55555555555556e-05 2.1792610397445e-10 84024.278965971 -209983.052384401;-2.77777777777778e-05 2.18114375549579e-10 86218.563955394 -209091.653439394]  x2=[-0.000694444444444444 9.18690500539298e-11 0 0;-0.000666666666666667 9.18062686265547e-11 0 0;-0.000638888888888889 9.17334196072622e-11 0 0;-0.000611111111111111 9.1650510984768e-11 0 0;-0.000583333333333333 9.15575518509369e-11 0 0;-0.000555555555555556 9.14545523997855e-11 58246.0351419008 -223856.455939284;-0.000527777777777778 9.13415239263644e-11 60587.012474446 -223234.242128182;-0.0005 9.12184788255193e-11 62921.3457583198 -222587.54816681;-0.000472222222222222 9.10854305905322e-11 65248.7790075721 -221916.444972447;-0.000444444444444444 9.09423938116413e-11 67569.0569929193 -221221.006139122;-0.000416666666666667 9.07893841744413e-11 69881.9252697332 -220501.30792954;-0.000388888888888889 9.06264184581633e-11 72187.1302059435 -219757.42926672;-0.000361111111111111 9.04535145338344e-11 74484.4190098517 -218989.451725339;-0.000333333333333333 9.02706913623184e-11 76773.5397578524 -218197.45952279;-0.000305555555555556 9.00779689922363e-11 79054.2414220595 -217381.539509942;-0.000277777777777778 8.98753685577677e-11 81326.2738978343 -216541.78116162;-0.00025 8.96629122763335e-11 83589.3880312124 -215678.276566789;-0.000222222222222222 8.9440623446159e-11 85843.3356462261 -214791.120418459;-0.000194444444444444 8.92085264437193e-11 88087.8695721197 -213880.4100033;-0.000166666666666667 8.89666467210664e-11 90322.7436704547 -212946.24519097;-0.000138888888888889 8.87150108030376e-11 92547.7128621014 -211988.72842317;-0.000111111111111111 8.84536462843469e-11 94762.5331541149 -211007.964702401;-8.33333333333333e-05 8.81825818265591e-11 96966.9616664913 -210004.06158046;-5.55555555555556e-05 8.79018471549467e-11 99160.7566588026 -208977.129146636;-2.77777777777778e-05 8.76114730552299e-11 101343.677556706 -207927.280015642]  x3=[-0.000694444444444444 3.13361138621949e-13 0 0;-0.000666666666666667 3.10033153370765e-13 0 0;-0.000638888888888889 3.06671169490557e-13 0 0;-0.000611111111111111 3.03275555660745e-13 0 0;-0.000583333333333333 2.9984668424865e-13 0 0;-0.000555555555555556 2.96384931268662e-13 60.6319356683411 -666.933123020829;-0.000527777777777778 2.92890676341006e-13 67.6125851665715 -666.261634393472;-0.0005 2.89364302650111e-13 74.5858201829138 -665.517082669817;-0.000472222222222222 2.85806196902591e-13 81.5508760235673 -664.699549498352;-0.000444444444444444 2.82216749284838e-13 88.50698889167 -663.809124530801;-0.000416666666666667 2.78596353420232e-13 95.4533959710575 -662.845905412296;-0.000388888888888889 2.74945406325978e-13 102.389335509915 -661.809997770669;-0.000361111111111111 2.71264308369567e-13 109.314046904311 -660.701515204865;-0.000333333333333333 2.67553463224873e-13 116.226770781606 -659.52057927249;-0.000305555555555556 2.63813277827882e-13 123.126749083728 -658.267319476476;-0.000277777777777778 2.60044162332072e-13 130.013225150302 -656.941873250883;-0.00025 2.56246530063431e-13 136.885443801621 -655.544385945826;-0.000222222222222222 2.52420797475133e-13 143.742651421469 -654.075010811536;-0.000194444444444444 2.48567384101868e-13 150.584096039756 -652.533908981555;-0.000166666666666667 2.44686712513836e-13 157.409027414984 -650.921249455066;-0.000138888888888889 2.40779208270408e-13 164.216697116517 -649.237209078358;-0.000111111111111111 2.36845299873459e-13 171.006358606658 -647.481972525436;-8.33333333333333e-05 2.32885418720374e-13 177.77726732251 -645.655732277769;-5.55555555555556e-05 2.28899999056747e-13 184.528680757633 -643.758688603178;-2.77777777777778e-05 2.24889477928754e-13 191.259858543462 -641.791049533881]  x4=[-0.000694444444444444 -4.15051450389667e-13 0 0;-0.000666666666666667 -4.08860673817014e-13 0 0;-0.000638888888888889 -4.02625061064035e-13 0 0;-0.000611111111111111 -3.96345295935939e-13 0 0;-0.000583333333333333 -3.90022067079737e-13 0 0;-0.000555555555555556 -3.83656067908732e-13 60.8630829248714 -352.170821952092;-0.000527777777777778 -3.77247996526469e-13 64.5475842975302 -351.514165236883;-0.0005 -3.70798555650188e-13 68.2250073001856 -350.818961032251;-0.000472222222222222 -3.64308452533761e-13 71.8949486619646 -350.085285575171;-0.000444444444444444 -3.5777839889013e-13 75.5570059324405 -349.313219321426;-0.000416666666666667 -3.51209110813265e-13 79.2107775257657 -348.50284693678;-0.000388888888888889 -3.44601308699632e-13 82.8558627647109 -347.654257287697;-0.000361111111111111 -3.37955717169196e-13 86.4918619246032 -346.767543431595;-0.000333333333333333 -3.31273064985958e-13 90.1183762771609 -345.842802606641;-0.000305555555555556 -3.24554084978036e-13 93.7350081342179 -344.880136221087;-0.000277777777777778 -3.17799513957304e-13 97.3413608913355 -343.87964984215;-0.00025 -3.11010092638592e-13 100.937039071294 -342.841453184437;-0.000222222222222222 -3.04186565558457e-13 104.521648367461 -341.76566009791;-0.000194444444444444 -2.97329680993537e-13 108.094795687033 -340.652388555404;-0.000166666666666667 -2.90440190878495e-13 111.65608919414 -339.50176063969;-0.000138888888888889 -2.8351885072356e-13 115.205138352817 -338.313902530084;-0.000111111111111111 -2.76566419531676e-13 118.74155396983 -337.088944488615;-8.33333333333333e-05 -2.69583659715271e-13 122.264948237355 -335.827020845736;-5.55555555555556e-05 -2.62571337012645e-13 125.774934775504 -334.528269985594;-2.77777777777778e-05 -2.55530220404007e-13 129.271128674701 -333.192834330857]  x5=0.000687048688231045  V1=[3.258e-10 2.261e+05 2.261e+05;377 377 377;2.369 0.194 -1.377]  V2=[4.31e-10 2.313e+05 2.313e+05;377 377 377;2.502 0.2568 -1.314]  I1=[9.177e-13 670.6 670.6;377 377 377;2.076 0.09296 -1.478]  I2=[4.71e-13 356.3 356.3;377 377 377;-2.438 0.173 -1.398]  nHarmo=1  Measurements=None
  Fault : powerlib/Elements/Three-Phase Fault  Commented=on  InitialStates=0  FaultA=on  FaultB=off  FaultC=off  GroundFault=on  SwitchTimes=1  External=off  SwitchStatus=NaN  FaultResistance=1e-9  GroundResistance=0.01  SnubberResistance=1e6  SnubberCapacitance=inf  Measurements=None
  Linear Transformer1 : powerlib/Elements/Linear Transformer  UNITS=pu  NominalPower=[ 150e8 60 ]  winding1="[ 230e3  0.002  0.08 ]"  winding2="[ 230e3  0.002  0.08 ]"  ThreeWindings=off  winding3=[3.15e+05 0.002 0.079997]  RmLm=[499.99 500]  Measurements=None  DataType=off
  Linear Transformer2 : powerlib/Elements/Linear Transformer  UNITS=pu  NominalPower=[ 150e8 60 ]  winding1="[ 230e3  0.002  0.08 ]"  winding2="[ 230e3  0.002  0.08 ]"  ThreeWindings=off  winding3=[3.15e+05 0.002 0.079997]  RmLm=[499.99 500]  Measurements=None  DataType=off
  Linear Transformer3 : powerlib/Elements/Linear Transformer  UNITS=pu  NominalPower=[ 150e8 60 ]  winding1="[ 230e3  0.002  0.08 ]"  winding2="[ 230e3  0.002  0.08 ]"  ThreeWindings=off  winding3=[3.15e+05 0.002 0.079997]  RmLm=[499.99 500]  Measurements=None  DataType=off
  Mimic Filter & Sampling : Subsystem
  Relay : Subsystem
  Scope : Scope  NumInputPorts=3
  Voltage Measurement Algorithm : Subsystem
  powergui : powerlib/powergui  Priority=1  SimulationMode=Discrete  SampleTime=1/1200/30  frequency=60  Iterations=50  frequencyindice=60  Pbase=100e6  ErrMax=0.0001  UnitsV=kV  UnitsW=MW  buscounter=0  FunctionMessages=off  echomessages=off  EnableUseOfTLC=off  CurrentSourceSwitches=off  DisableSnubberDevices=off  DisableRonSwitches=off  DisableVfSwitches=off  DisplayEquations=off  AutomaticDiscreteSolvers=off  SolverType=Tustin/Backward Euler (TBE)  Interpol=off  ExternalGateDelay=off  methode=off  Ts=100  x0status=blocks  SPID=on  SwTol=0  HookPort=off  NonlinearTolerance=1e-4  nMaxIteration=100  ContinueOnMaxIteration=off  RestoreLinks=warning  ResistiveCurrentMeasurement=off  Frange=[0:2:500]  Ylog=off  Xlog=on  ShowGrid=off  save=off  variable=ZData  structure=0  ZoomFFT=off  StartTime=0.0  cycles=1  DisplayStyle=1  fundamental=60  FreqAxis=off  MaxFrequency=1000  frequencyindicesteady=1  RmsSteady=1  display=off
  tag scope: Ia=global, Ib=global, Ic=global
  wires:
  Mimic Filter & Sampling/1(Ia) -> Scope/1, [Ia]
  Mimic Filter & Sampling/2(Ib) -> Scope/2, [Ib]
  Mimic Filter & Sampling/3(Ic) -> Scope/3, [Ic]
  connections:
  Distributed Parameters Line3/LConn2 -- Distributed Parameters Line1/RConn2 -- 100+j35 MVA/LConn2 -- Fault/LConn2
  Distributed Parameters Line3/LConn3 -- Fault/LConn3 -- Distributed Parameters Line1/RConn3 -- 100+j35 MVA/LConn3
  Distributed Parameters Line5/RConn1 -- Distributed Parameters Line8/LConn1 -- 90+j30 MVA/LConn1
  Distributed Parameters Line5/RConn3 -- Distributed Parameters Line8/LConn3 -- 90+j30 MVA/LConn3
  Distributed Parameters Line6/LConn1 -- Distributed Parameters Line7/LConn1 -- 125+j50 MVA/LConn1
  Distributed Parameters Line6/LConn2 -- Distributed Parameters Line7/LConn2 -- 125+j50 MVA/LConn2
  Distributed Parameters Line6/LConn3 -- Distributed Parameters Line7/LConn3 -- 125+j50 MVA/LConn3
  Distributed Parameters Line3/RConn1 -- 13.8 KV/230 KV 5.86 %Z/RConn1 -- Distributed Parameters Line8/RConn1
  Distributed Parameters Line3/RConn2 -- 13.8 KV/230 KV 5.86 %Z/RConn2 -- Distributed Parameters Line8/RConn2
  Distributed Parameters Line3/RConn3 -- 13.8 KV/230 KV 5.86 %Z/RConn3 -- Distributed Parameters Line8/RConn3
  18KV/230KV 6.25 %Z/RConn1 -- Relay/LConn1 -- Distributed Parameters Line7/RConn1
  18KV/230KV 6.25 %Z/RConn2 -- Relay/LConn2 -- Distributed Parameters Line7/RConn2
  18KV/230KV 6.25 %Z/RConn3 -- Relay/LConn3 -- Distributed Parameters Line7/RConn3
  Distributed Parameters Line5/RConn2 -- Distributed Parameters Line8/LConn2 -- 90+j30 MVA/LConn2
  Distributed Parameters Line6/RConn1 -- "16.5 KV/230 KV 5.76 %Z     "/RConn1 -- Distributed Parameters Line5/LConn1
  Distributed Parameters Line6/RConn2 -- "16.5 KV/230 KV 5.76 %Z     "/RConn2 -- Distributed Parameters Line5/LConn2
  Distributed Parameters Line6/RConn3 -- "16.5 KV/230 KV 5.76 %Z     "/RConn3 -- Distributed Parameters Line5/LConn3
  247.5 MW/RConn1 -- "16.5 KV/230 KV 5.76 %Z     "/LConn1
  247.5 MW/RConn2 -- "16.5 KV/230 KV 5.76 %Z     "/LConn2
  247.5 MW/RConn3 -- "16.5 KV/230 KV 5.76 %Z     "/LConn3
  128 MW/RConn1 -- 13.8 KV/230 KV 5.86 %Z/LConn1
  128 MW/RConn2 -- 13.8 KV/230 KV 5.86 %Z/LConn2
  128 MW/RConn3 -- 13.8 KV/230 KV 5.86 %Z/LConn3
  192 MW/RConn1 -- 18KV/230KV 6.25 %Z/LConn1
  192 MW/RConn2 -- 18KV/230KV 6.25 %Z/LConn2
  192 MW/RConn3 -- 18KV/230KV 6.25 %Z/LConn3
  Mimic Filter & Sampling/LConn1 -- Linear Transformer2/RConn1
  Mimic Filter & Sampling/LConn2 -- Linear Transformer2/RConn2
  Linear Transformer1/RConn1 -- Mimic Filter & Sampling/LConn3
  Linear Transformer1/RConn2 -- Mimic Filter & Sampling/LConn4
  Linear Transformer3/RConn1 -- Mimic Filter & Sampling/LConn5
  Linear Transformer3/RConn2 -- Mimic Filter & Sampling/LConn6
  100+j35 MVA/LConn1 -- Fault/LConn1 -- Distributed Parameters Line1/RConn1 -- Distributed Parameters Line3/LConn1
  Linear Transformer2/LConn1 -- Relay/RConn1
  Linear Transformer2/LConn2 -- Distributed Parameters Line1/LConn1
  Linear Transformer1/LConn1 -- Relay/RConn2
  Linear Transformer1/LConn2 -- Distributed Parameters Line1/LConn2
  Linear Transformer3/LConn1 -- Relay/RConn3
  Linear Transformer3/LConn2 -- Distributed Parameters Line1/LConn3

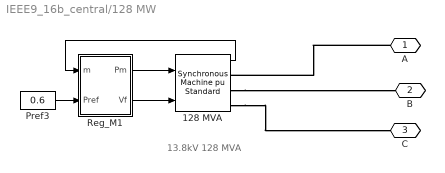
== system IEEE9_16b_central/128 MW ==
  note: 13.8kV 128 MVA
  128 MVA : powerlib/Machines/Synchronous Machine pu Standard  PresetModel=No  MechanicalLoad=Mechanical power Pm  ShowDetailedParameters=on  RotorType=Salient-pole  Units=per unit standard parameters  MeasurementBus=off  NominalParameters="[128e6  13800   60 ]"  Reactances1=[ 31 32 33 34 35 36 37 ]  Reactances2=[ 1.305, 0.296, 0.252, 0.474, 0.243, 0.18 ]  dAxisTimeConstants=Short-circuit  qAxisTimeConstants=Open-circuit  TimeConstants1=[]  TimeConstants2=[]  TimeConstants3=[]  TimeConstants4=[]  TimeConstants5=[ 1.01, 0.053, 0.1 ]  TimeConstants6=[]  TimeConstants7=[]  TimeConstants8=[]  StatorResistance=2.8544e-3  Mechanical="[20 0  32]"  PolePairs=32  InitialConditions=[0 -74.5248 0.603223 0.603223 0.603223 5.08525 -114.915 125.085 1.10339]  SetSaturation=off  Saturation=[0.6404,0.7127,0.8441,0.9214,0.9956,1.082,1.19,1.316,1.457;0.7,0.7698,0.8872,0.9466,0.9969,1.046,1.1,1.151,1.201]  LoadFlowParameters=[1 500000000 0 0 0]  TsPowergui=0  TsBlock=-1  IterativeModel=Trapezoidal non iterative  IterativeDiscreteModel=Trapezoidal non iterative  BusType=PV  Pref=0.6*128e6  Qref=0  Qmin=-Inf  Qmax=Inf  PLF=0  QLF=0
      settings: AttributesFormatString=\n\n
  Pref3 : Constant  Value=0.6
  Reg_M1 : Subsystem
  A : PMIOPort  Side=Right
  B : PMIOPort  Port=2  Side=Right
  C : PMIOPort  Port=3  Side=Right
  wires:
  Reg_M1/1(Pm) -> 128 MVA/1
  Reg_M1/2(Vf) -> 128 MVA/2
  Pref3/1 -> Reg_M1/2(Pref)
  128 MVA/1 -> Reg_M1/1(m)
  connections:
  A/RConn1 -- 128 MVA/RConn1
  128 MVA/RConn2 -- B/RConn1
  128 MVA/RConn3 -- C/RConn1
